simulink model "lab_7_task_3_simulink"  (R2025b)
settings: Solver=ode4  StartTime=0.0  StopTime=10.0  FixedStep=0.0001  RelTol=1e-3
values from neighbouring files (symbols this model uses):
  a = 7093    [lab_7_task_1.m]    (also in lab_7_task_2.m; lab_7_task_3.m; lab_7_task_4.m; project_review.m)
  A_BN0 = eye(3)    [lab_7_task_1.m]    (also in lab_7_task_3.m; lab_7_task_4.m; project_review.m)
  area = [ ... (first row only)    [lab_7_task_3.m]    (also in lab_7_task_4.m; project_review.m)
  e = 0.5    [lab_7_task_1.m]    (also in lab_7_task_2.m; lab_7_task_3.m = 0.00277; lab_7_task_4.m = 0.00277; project_review.m = 0.00277)
  e_sun = deg2rad(23.45)    [lab_7_task_1.m]    (also in lab_7_task_2.m; lab_7_task_3.m; lab_7_task_4.m; project_review.m)
  I = diag([ix iy iz])    [lab_4_task_1.m]    (also in lab_5_task_1.m; lab_5_task_2.m; lab_6_task_1.m = diag([ ix iy iz ]); lab_6_task_2.m = diag([ ix iy iz ]))
  inc = deg2rad(98.27)    [lab_7_task_1.m]    (also in lab_7_task_2.m; lab_7_task_3.m; lab_7_task_4.m; project_review.m = deg2rad(20))
  mu = astroConstants(13)    [lab_7_task_3.m]    (also in lab_7_task_4.m; project_review.m = 398345.74)
  n = sqrt(G*M_e/R^3)    [lab_6_task_1.m]    (also in lab_6_task_2.m; lab_7_task_1.m = sqrt(mu_E/(a^3)); lab_7_task_2.m = sqrt(mu_E/(a^3)); lab_7_task_3.m = sqrt(mu/(a^3)))
  N_B = [ ... (first row only)    [lab_7_task_3.m]    (also in lab_7_task_4.m; project_review.m)
  n_sun = 2*pi / (60*60*24*365)    (= 1.99238499086e-07)    [lab_7_task_1.m]    (also in lab_7_task_2.m; lab_7_task_3.m; lab_7_task_4.m = 1.99102127766e-07; project_review.m = 1.99102127766e-07)
  P = F_e / c    (= 4.52968645764e-06)    [lab_7_task_3.m]    (also in lab_7_task_4.m; project_review.m)
  r_Fi = [ ... (first row only)    [lab_7_task_3.m]    (also in lab_7_task_4.m; project_review.m)
  r_sun = 1.496e8    (= 149600000)    [lab_7_task_1.m]    (also in lab_7_task_2.m; lab_7_task_3.m; lab_7_task_4.m; project_review.m)
  rho_d = [0.1 0.1 0.1 0.1 0.1 0.1      0.1 0.1 0.1 0.1]    [lab_7_task_3.m]    (also in lab_7_task_4.m; project_review.m)
  rho_s = [0.5 0.5 0.5 0.5 0.5 0.5      0.1 0.1 0.1 0.1]    [lab_7_task_3.m]    (also in lab_7_task_4.m; project_review.m)
  TA0 = deg2rad(0)    [lab_7_task_1.m]    (also in lab_7_task_2.m; lab_7_task_3.m; lab_7_task_4.m; project_review.m)
undefined symbols (not defined in the file or in its folder): i
libraries: vec_norm x2, dynamics x1, matrix_library x1
settings Model: VariantFading=off  Creator=nicol  LastModifiedBy=nicol

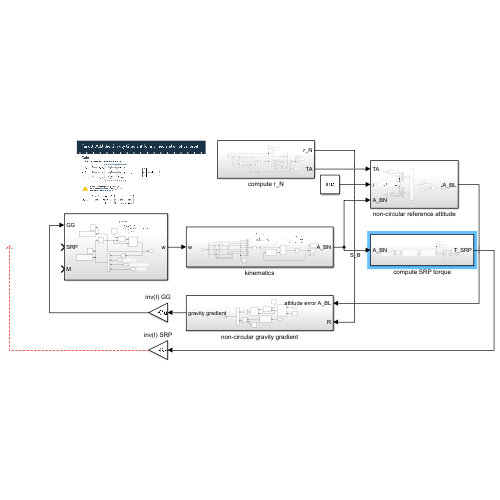
[thumbnail: Simulink's stored preview of the top-level diagram]
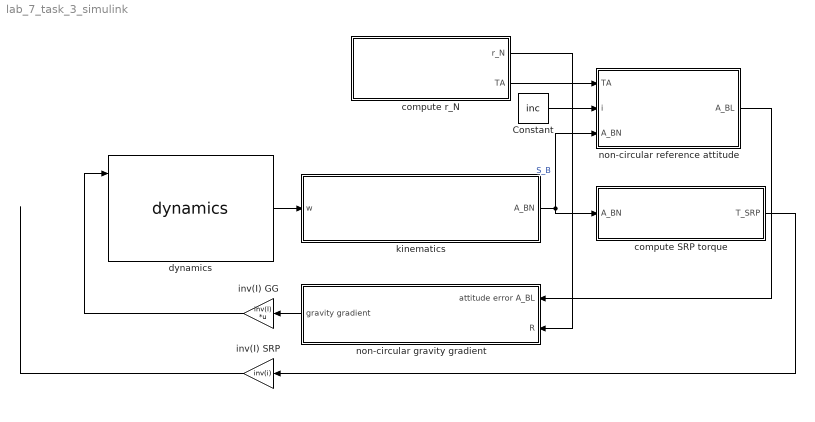
== system lab_7_task_3_simulink ==
  Constant : Constant  Value=inc
  compute SRP torque : Subsystem
  compute r_N : Subsystem
  dynamics : dynamics/dynamics  SystemSampleTime=-1  VariantActivationTime=update diagram  EmptyChoice=off  PassThrough=off  PassThroughVariantControl=(default)  EmptyChoiceVariantControl=(default)  AllowFlexibleInterface=on  Latency=0  AutoFrameSizeCalculation=off
  inv(I) GG : Gain  Gain=inv(I)  Multiplication=Matrix(K*u)
  inv(I) SRP : Gain  Gain=inv(i)
  kinematics : Subsystem
  non-circular gravity gradient : Subsystem
      settings: PortSchema="{\"entries\":[{\"content\":{\"sides\":[{\"content\":{\"connectorIds\":[\"Out1\"]},\"type\":\"ConnectorPlacement.EquallySpacedRectSide\",\"uuid\":\"2a67419a-68c9-4369-a698-e6ac26417455\"},{\"content\":{\"connectorIds\":[\"In1\",\"In2\"],\"side\":\"RIGHT\"},\"type\":\"ConnectorPlacement.EquallySpacedRectSide\",\"uuid\":\"5f3f4c4a-6b79-4b92-8f4c-19ffa36753b2\"},{\"content\":{\"side\":\"TOP\"},\"type\":\"ConnectorPlacement.EquallySpacedRectSide\",\"uuid\":\"22c946b7-ea77-4444-a63c-d5b3d585f671\"}]},\"type\":\"ConnectorPlacement.EquallySpacedConnector\",\"uuid\":\"037c4a72-b28b-418e-a921-9da68dc0cd93\"}],\"packageUris\":[\"http://schema.mathworks.com/mf0/Connector/R2020b\"],\"version\":\"1.0\"}"
  non-circular reference attitude : Subsystem
  wires:
  compute r_N/1(r_N) -> non-circular gravity gradient/2(R)
  Constant/1 -> non-circular reference attitude/2(i)
  inv(I) GG/1 -> dynamics/1
  compute r_N/2(TA) -> non-circular reference attitude/1(TA)
  dynamics/1 -> kinematics/1(w)
  kinematics/1(A_BN) -> compute SRP torque/1(A_BN), non-circular reference attitude/3(A_BN)  "S_B"
  non-circular reference attitude/1(A_BL) -> non-circular gravity gradient/1(attitude error A_BL)
  compute SRP torque/1(T_SRP) -> inv(I) SRP/1
  inv(I) SRP/1 -> ?
  non-circular gravity gradient/1(gravity gradient) -> inv(I) GG/1

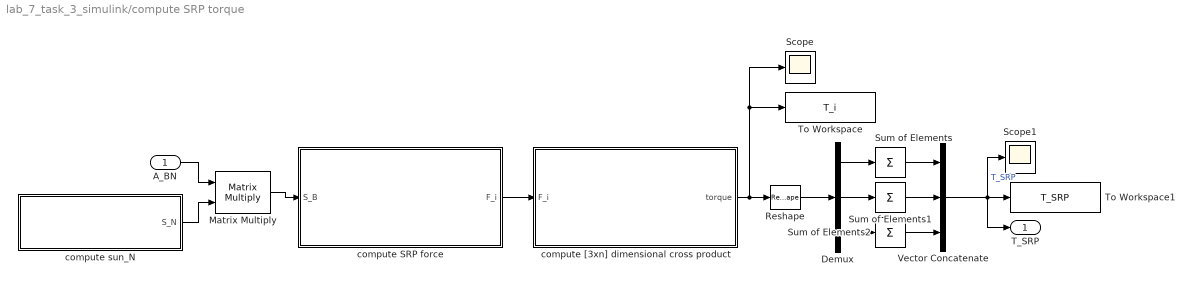
== system lab_7_task_3_simulink/compute SRP torque ==
  A_BN : Inport
  Demux : Demux  Outputs=3
  Matrix Multiply : Product  Multiplication=Matrix(*)
  Reshape : Reshape
  Scope : Scope
      settings: ActiveDisplayYMinimum=-1  ActiveDisplayYMaximum=1  DataLoggingVariableName=ScopeData6
  Scope1 : Scope
      settings: ActiveDisplayYMinimum=-2.7188018298935311E-7  ActiveDisplayYMaximum=4.8585990784799191E-7  DataLoggingVariableName=ScopeData7
  Sum of Elements : Sum  Inputs=+
  Sum of Elements1 : Sum  Inputs=+
  Sum of Elements2 : Sum  Inputs=+
  To Workspace : ToWorkspace  VariableName=T_i  SaveFormat=Timeseries  SampleTime=-1
  To Workspace1 : ToWorkspace  VariableName=T_SRP  SaveFormat=Timeseries  SampleTime=-1
  Vector Concatenate : Concatenate  NumInputs=3
  compute SRP force : Subsystem
  compute [3xn] dimensional cross product : Subsystem
  compute sun_N : Subsystem
  T_SRP : Outport
  wires:
  Matrix Multiply/1 -> compute SRP force/1(S_B)
  compute [3xn] dimensional cross product/1(torque) -> Scope/1, To Workspace/1, Reshape/1
  compute SRP force/1(F_i) -> compute [3xn] dimensional cross product/1(F_i)
  compute sun_N/1(S_N) -> Matrix Multiply/2
  A_BN/1 -> Matrix Multiply/1
  Reshape/1 -> Demux/1
  Demux/3 -> Sum of Elements2/1
  Demux/2 -> Sum of Elements1/1
  Demux/1 -> Sum of Elements/1
  Sum of Elements1/1 -> Vector Concatenate/2
  Sum of Elements/1 -> Vector Concatenate/1
  Sum of Elements2/1 -> Vector Concatenate/3
  Vector Concatenate/1 -> T_SRP/1, Scope1/1, To Workspace1/1  "T_SRP"

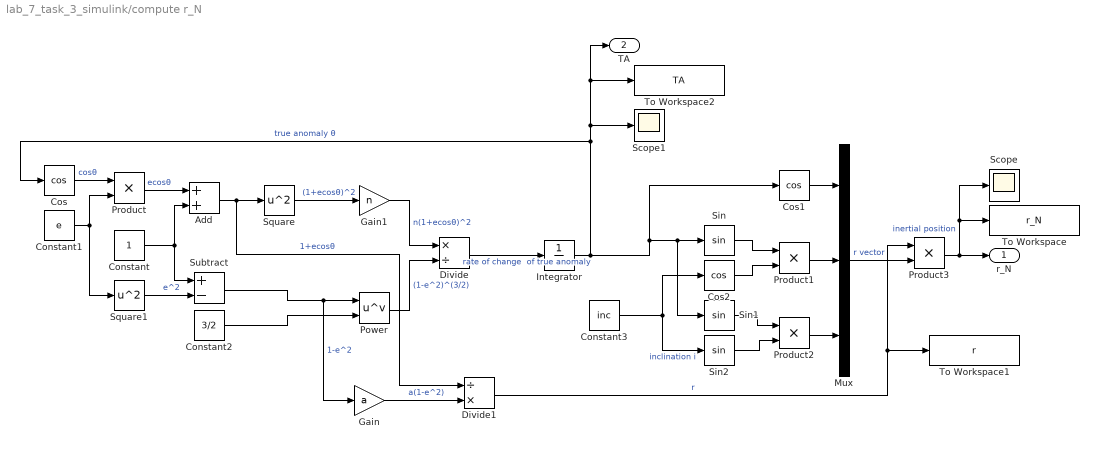
== system lab_7_task_3_simulink/compute r_N ==
  Add : Sum
  Constant : Constant
  Constant1 : Constant  Value=e
  Constant2 : Constant  Value=3/2
  Constant3 : Constant  Value=inc
  Cos : Trigonometry  Operator=cos
  Cos1 : Trigonometry  Operator=cos
  Cos2 : Trigonometry  Operator=cos
  Divide : Product  Inputs=*/
  Divide1 : Product  Inputs=/*
  Gain : Gain  Gain=a
  Gain1 : Gain  Gain=n
  Integrator : Integrator  InitialCondition=TA0
  Mux : Mux  Inputs=3
  Power : Math  Operator=pow
  Product{,1..3} (4 alike) : Product
  Scope : Scope
      settings: ActiveDisplayYMinimum=-1  ActiveDisplayYMaximum=1  DataLoggingVariableName=ScopeData3
  Scope1 : Scope
      settings: ActiveDisplayYMinimum=-1  ActiveDisplayYMaximum=1  DataLoggingVariableName=ScopeData5
  Sin : Trigonometry
  Sin1 : Trigonometry
  Sin2 : Trigonometry
  Square : Math  Operator=square
  Square1 : Math  Operator=square
  Subtract : Sum  Inputs=+-
  To Workspace : ToWorkspace  VariableName=r_N  SaveFormat=Timeseries  SampleTime=-1
  To Workspace1 : ToWorkspace  VariableName=r  SaveFormat=Timeseries  SampleTime=-1
  To Workspace2 : ToWorkspace  VariableName=TA  SaveFormat=Timeseries  SampleTime=-1
  r_N : Outport
  TA : Outport  Port=2
  wires:
  Integrator/1 -> Sin1/1, Sin/1, Cos1/1, To Workspace2/1, TA/1, Scope1/1, Cos/1  "true anomaly θ"
  Add/1 -> Divide1/1, Square/1  "1+ecosθ"
  Square/1 -> Gain1/1  "(1+ecosθ)^2"
  Gain1/1 -> Divide/1  "n(1+ecosθ)^2"
  Sin1/1 -> Product2/1
  Constant/1 -> Subtract/1, Add/2
  Subtract/1 -> Gain/1, Power/1  "1-e^2"
  Product3/1 -> r_N/1, To Workspace/1, Scope/1  "inertial position"
  Constant3/1 -> Cos2/1, Sin2/1  "inclination i"
  Gain/1 -> Divide1/2  "a(1-e^2)"
  Constant2/1 -> Power/2
  Sin2/1 -> Product2/2
  Cos/1 -> Product/1  "cosθ"
  Constant1/1 -> Square1/1, Product/2
  Product/1 -> Add/1  "ecosθ"
  Product2/1 -> Mux/3
  Square1/1 -> Subtract/2  "e^2"
  Divide1/1 -> Product3/1, To Workspace1/1  "r"
  Cos1/1 -> Mux/1
  Mux/1 -> Product3/2  "r vector"
  Power/1 -> Divide/2  "(1-e^2)^(3/2)"
  Product1/1 -> Mux/2
  Divide/1 -> Integrator/1  "rate of change  of true anomaly"
  Sin/1 -> Product1/1
  Cos2/1 -> Product1/2

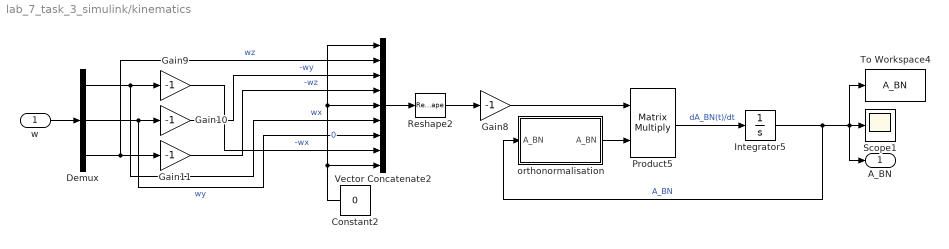
== system lab_7_task_3_simulink/kinematics ==
  w : Inport
  Constant2 : Constant  Value=0
  Demux : Demux  Outputs=3
  Gain{8..11} (4 alike) : Gain  Gain=-1
  Integrator5 : Integrator  InitialCondition=A_BN0
  Product5 : Product  Multiplication=Matrix(*)
  Reshape2 : Reshape  OutputDimensionality=Customize  OutputDimensions=[3,3]
  Scope1 : Scope
      settings: ActiveDisplayYMinimum=-1.2499999998899596  ActiveDisplayYMaximum=1.2499999999877733
  To Workspace4 : ToWorkspace  VariableName=A_BN  SaveFormat=Timeseries  SampleTime=-1
  Vector Concatenate2 : Concatenate  NumInputs=9
  orthonormalisation : Subsystem
  A_BN : Outport
  wires:
  Product5/1 -> Integrator5/1  "dA_BN(t)/dt"
  Gain11/1 -> Vector Concatenate2/4  "-wz"
  Integrator5/1 -> A_BN/1, To Workspace4/1, Scope1/1, orthonormalisation/1(A_BN)  "A_BN"
  Gain8/1 -> Product5/1
  Demux/1 -> Vector Concatenate2/6, Gain9/1  "wx"
  Reshape2/1 -> Gain8/1
  Gain10/1 -> Vector Concatenate2/3  "-wy"
  Demux/2 -> Vector Concatenate2/7, Gain10/1  "wy"
  Vector Concatenate2/1 -> Reshape2/1
  Demux/3 -> Vector Concatenate2/2, Gain11/1  "wz"
  Constant2/1 -> Vector Concatenate2/1, Vector Concatenate2/5, Vector Concatenate2/9  "0"
  Gain9/1 -> Vector Concatenate2/8  "-wx"
  w/1 -> Demux/1
  orthonormalisation/1(" A_BN") -> Product5/2

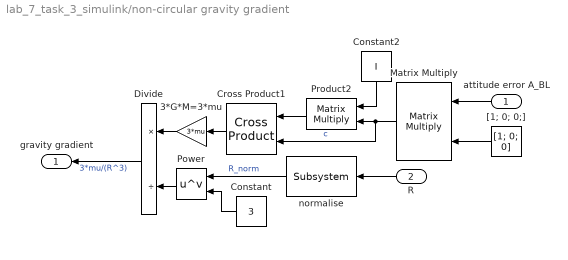
== system lab_7_task_3_simulink/non-circular gravity gradient ==
  attitude error A_BL : Inport
  R : Inport  Port=2
  3*G*M=3*mu : Gain  Gain=3*mu
  Constant : Constant  Value=3
  Constant2 : Constant  Value=I
  Cross Product1 : matrix_library/Cross Product
  Divide : Product  Inputs=*/
  Matrix Multiply : Product  Multiplication=Matrix(*)
  Power : Math  Operator=pow
  Product2 : Product  Multiplication=Matrix(*)
  "[1; 0; 0;]" : Constant  Value=[1; 0; 0]
  normalise : vec_norm/Subsystem  SystemSampleTime=-1  VariantActivationTime=update diagram  EmptyChoice=off  PassThrough=off  PassThroughVariantControl=(default)  EmptyChoiceVariantControl=(default)  AllowFlexibleInterface=on  Latency=0  AutoFrameSizeCalculation=off
  gravity gradient : Outport
  wires:
  Matrix Multiply/1 -> Cross Product1/2, Product2/2  "c"
  attitude error A_BL/1 -> Matrix Multiply/1
  Constant2/1 -> Product2/1
  Cross Product1/1 -> 3*G*M=3*mu/1
  Product2/1 -> Cross Product1/1
  "[1; 0; 0;]"/1 -> Matrix Multiply/2
  3*G*M=3*mu/1 -> Divide/1
  Divide/1 -> gravity gradient/1  "3*mu/(R^3)"
  R/1 -> normalise/1
  Constant/1 -> Power/2
  Power/1 -> Divide/2
  normalise/1 -> Power/1  "R_norm"

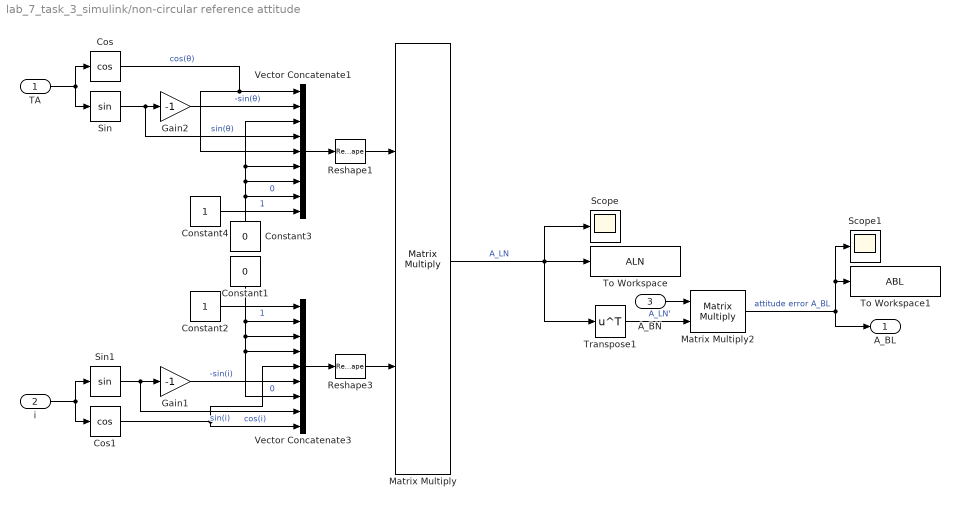
== system lab_7_task_3_simulink/non-circular reference attitude ==
  TA : Inport
  i : Inport  Port=2
  A_BN : Inport  Port=3
  Constant1 : Constant  Value=0
  Constant2 : Constant
  Constant3 : Constant  Value=0
  Constant4 : Constant
  Cos : Trigonometry  Operator=cos
  Cos1 : Trigonometry  Operator=cos
  Gain1 : Gain  Gain=-1
  Gain2 : Gain  Gain=-1
  Matrix Multiply : Product  Multiplication=Matrix(*)
  Matrix Multiply2 : Product  Multiplication=Matrix(*)
  Reshape1 : Reshape  OutputDimensionality=Customize  OutputDimensions=[3,3]
  Reshape3 : Reshape  OutputDimensionality=Customize  OutputDimensions=[3,3]
  Scope : Scope
      settings: ActiveDisplayYMinimum=-1.2499999999912785  ActiveDisplayYMaximum=1.249999999999031  DataLoggingVariableName=ScopeData2
  Scope1 : Scope
      settings: ActiveDisplayYMinimum=-1  ActiveDisplayYMaximum=1  DataLoggingVariableName=ScopeData4
  Sin : Trigonometry
  Sin1 : Trigonometry
  To Workspace : ToWorkspace  VariableName=ALN  SaveFormat=Timeseries  SampleTime=-1
  To Workspace1 : ToWorkspace  VariableName=ABL  SaveFormat=Timeseries  SampleTime=-1
  Transpose1 : Math  Operator=transpose
  Vector Concatenate1 : Concatenate  NumInputs=9
  Vector Concatenate3 : Concatenate  NumInputs=9
  A_BL : Outport
  wires:
  Constant3/1 -> Vector Concatenate1/8, Vector Concatenate1/7, Vector Concatenate1/6, Vector Concatenate1/3  "0"
  TA/1 -> Sin/1, Cos/1
  Gain2/1 -> Vector Concatenate1/2  "-sin(θ)"
  Sin/1 -> Vector Concatenate1/4, Gain2/1  "sin(θ)"
  Matrix Multiply/1 -> Scope/1, Transpose1/1, To Workspace/1  "A_LN"
  Cos/1 -> Vector Concatenate1/5, Vector Concatenate1/1  "cos(θ)"
  Vector Concatenate1/1 -> Reshape1/1
  Constant4/1 -> Vector Concatenate1/9  "1"
  Transpose1/1 -> Matrix Multiply2/2  "A_LN'"
  Reshape1/1 -> Matrix Multiply/1
  Reshape3/1 -> Matrix Multiply/2
  Vector Concatenate3/1 -> Reshape3/1
  Cos1/1 -> Vector Concatenate3/5, Vector Concatenate3/9  "cos(i)"
  Sin1/1 -> Vector Concatenate3/8, Gain1/1  "sin(i)"
  i/1 -> Sin1/1, Cos1/1
  Constant1/1 -> Vector Concatenate3/7, Vector Concatenate3/4, Vector Concatenate3/3, Vector Concatenate3/2  "0"
  Constant2/1 -> Vector Concatenate3/1  "1"
  Gain1/1 -> Vector Concatenate3/6  "-sin(i)"
  A_BN/1 -> Matrix Multiply2/1
  Matrix Multiply2/1 -> Scope1/1, To Workspace1/1, A_BL/1  "attitude error A_BL"

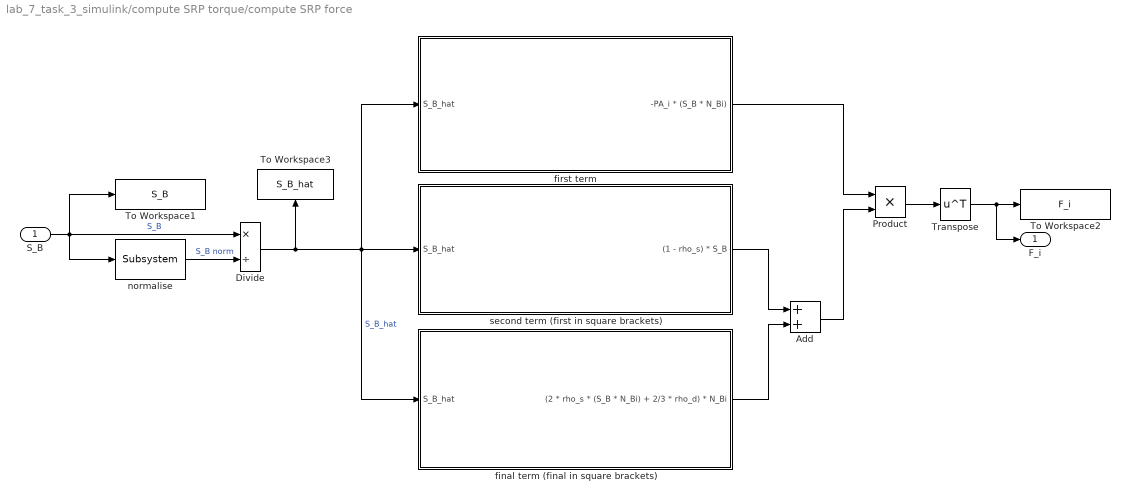
== system lab_7_task_3_simulink/compute SRP torque/compute SRP force ==
  S_B : Inport
  Add : Sum
  Divide : Product  Inputs=*/
  Product : Product
  To Workspace1 : ToWorkspace  VariableName=S_B  SaveFormat=Timeseries  SampleTime=-1
  To Workspace2 : ToWorkspace  VariableName=F_i  SaveFormat=Timeseries  SampleTime=-1
  To Workspace3 : ToWorkspace  VariableName=S_B_hat  SaveFormat=Timeseries  SampleTime=-1
  Transpose : Math  Operator=transpose
  final term (final in square brackets) : Subsystem
  first term : Subsystem
  normalise : vec_norm/Subsystem  SystemSampleTime=-1  VariantActivationTime=update diagram  EmptyChoice=off  PassThrough=off  PassThroughVariantControl=(default)  EmptyChoiceVariantControl=(default)  AllowFlexibleInterface=on  Latency=0  AutoFrameSizeCalculation=off
  second term (first in square brackets) : Subsystem
  F_i : Outport
  wires:
  final term (final in square brackets)/1((2 * rho_s * (S_B * N_Bi) + 2/3 * rho_d) * N_Bi) -> Add/2
  Transpose/1 -> F_i/1, To Workspace2/1
  first term/1(-PA_i * (S_B * N_Bi)) -> Product/1
  Add/1 -> Product/2
  second term (first in square brackets)/1((1 - rho_s) * S_B) -> Add/1
  Product/1 -> Transpose/1
  normalise/1 -> Divide/2  "S_B norm"
  Divide/1 -> second term (first in square brackets)/1(S_B_hat), first term/1(S_B_hat), final term (final in square brackets)/1(S_B_hat), To Workspace3/1  "S_B_hat"
  S_B/1 -> normalise/1, Divide/1, To Workspace1/1  "S_B"

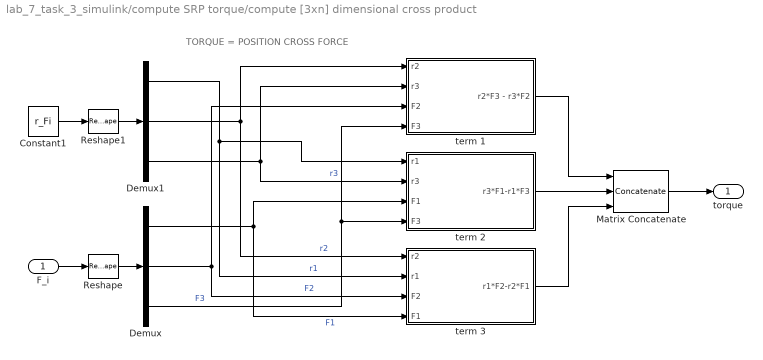
== system lab_7_task_3_simulink/compute SRP torque/compute [3xn] dimensional cross product ==
  note: TORQUE = POSITION CROSS FORCE
  F_i : Inport
  Constant1 : Constant  Value=r_Fi
  Demux : Demux  Outputs=3
  Demux1 : Demux  Outputs=3
  Matrix Concatenate : Concatenate  NumInputs=3  Mode=Multidimensional array  ConcatenateDimension=2
  Reshape : Reshape
  Reshape1 : Reshape
  term 1 : Subsystem
  term 2 : Subsystem
  term 3 : Subsystem
  torque : Outport
  wires:
  term 2/1(r3*F1-r1*F3) -> Matrix Concatenate/2
  Demux1/2 -> term 1/1(r2), term 3/1(r2)  "r2"
  term 3/1(r1*F2-r2*F1) -> Matrix Concatenate/3
  term 1/1(r2*F3 - r3*F2) -> Matrix Concatenate/1
  Demux/2 -> term 1/3(F2), term 3/3(F2)  "F2"
  Demux/3 -> term 1/4(F3), term 2/4(F3)  "F3"
  F_i/1 -> Reshape/1
  Demux1/3 -> term 1/2(r3), term 2/2(r3)  "r3"
  Reshape1/1 -> Demux1/1
  Constant1/1 -> Reshape1/1
  Demux/1 -> term 2/3(F1), term 3/4(F1)  "F1"
  Demux1/1 -> term 3/2(r1), term 2/1(r1)  "r1"
  Reshape/1 -> Demux/1
  Matrix Concatenate/1 -> torque/1

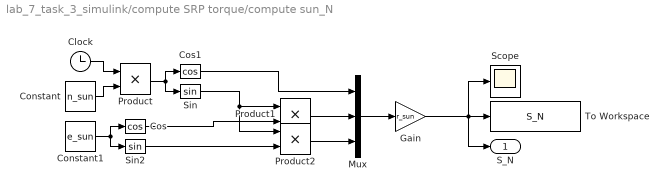
== system lab_7_task_3_simulink/compute SRP torque/compute sun_N ==
  Clock : Clock
  Constant : Constant  Value=n_sun
  Constant1 : Constant  Value=e_sun
  Cos : Trigonometry  Operator=cos
  Cos1 : Trigonometry  Operator=cos
  Gain : Gain  Gain=r_sun
  Mux : Mux  Inputs=3
  Product : Product
  Product1 : Product
  Product2 : Product
  Scope : Scope
      settings: ActiveDisplayYMinimum=-1.8699999999999996E+7  ActiveDisplayYMaximum=1.683E+8
  Sin : Trigonometry
  Sin2 : Trigonometry
  To Workspace : ToWorkspace  VariableName=S_N  SaveFormat=Timeseries  SampleTime=-1
  S_N : Outport
  wires:
  Constant/1 -> Product/2
  Clock/1 -> Product/1
  Product/1 -> Sin/1, Cos1/1
  Constant1/1 -> Sin2/1, Cos/1
  Cos1/1 -> Mux/1
  Product1/1 -> Mux/2
  Product2/1 -> Mux/3
  Sin/1 -> Product2/1, Product1/1
  Cos/1 -> Product1/2
  Sin2/1 -> Product2/2
  Gain/1 -> S_N/1, Scope/1, To Workspace/1
  Mux/1 -> Gain/1

== system lab_7_task_3_simulink/kinematics/orthonormalisation ==
  A_BN : Inport
  Gain : Gain  Gain=3/2
  Gain1 : Gain  Gain=1/2
  Matrix Multiply1 : Product  Inputs=3  Multiplication=Matrix(*)
  Subtract : Sum  Inputs=+-
  Transpose1 : Math  Operator=transpose
  " A_BN" : Outport
  wires:
  Gain/1 -> Subtract/1
  Transpose1/1 -> Matrix Multiply1/2
  Matrix Multiply1/1 -> Gain1/1
  Gain1/1 -> Subtract/2
  Subtract/1 -> " A_BN"/1
  A_BN/1 -> Matrix Multiply1/1, Gain/1, Transpose1/1, Matrix Multiply1/3

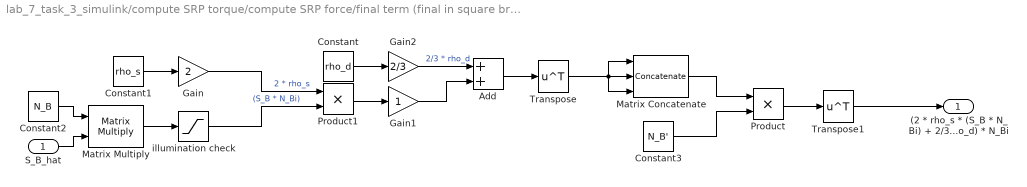
== system lab_7_task_3_simulink/compute SRP torque/compute SRP force/final term (final in square brackets) ==
  S_B_hat : Inport
  Add : Sum
  Constant : Constant  Value=rho_d
  Constant1 : Constant  Value=rho_s
  Constant2 : Constant  Value=N_B
  Constant3 : Constant  Value=N_B'
  Gain : Gain  Gain=2
  Gain1 : Gain
  Gain2 : Gain  Gain=2/3
  Matrix Concatenate : Concatenate  NumInputs=3  Mode=Multidimensional array
  Matrix Multiply : Product  Multiplication=Matrix(*)
  Product : Product
  Product1 : Product
  Transpose : Math  Operator=transpose
  Transpose1 : Math  Operator=transpose
  illumination check : Saturate  UpperLimit=inf  LowerLimit=0
  (2 * rho_s * (S_B * N_Bi) + 2/3 * rho_d) * N_Bi : Outport
  wires:
  Constant1/1 -> Gain/1
  Product1/1 -> Gain1/1
  Gain1/1 -> Add/2
  Transpose1/1 -> (2 * rho_s * (S_B * N_Bi) + 2/3 * rho_d) * N_Bi/1
  Constant3/1 -> Product/2
  Transpose/1 -> Matrix Concatenate/3, Matrix Concatenate/1, Matrix Concatenate/2
  S_B_hat/1 -> Matrix Multiply/2
  Constant2/1 -> Matrix Multiply/1
  Matrix Multiply/1 -> illumination check/1
  Gain/1 -> Product1/1  "2 * rho_s"
  Constant/1 -> Gain2/1
  Gain2/1 -> Add/1  "2/3 * rho_d"
  Add/1 -> Transpose/1
  Matrix Concatenate/1 -> Product/1
  Product/1 -> Transpose1/1
  illumination check/1 -> Product1/2  "(S_B * N_Bi)"

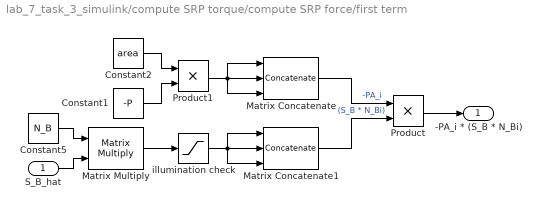
== system lab_7_task_3_simulink/compute SRP torque/compute SRP force/first term ==
  S_B_hat : Inport
  Constant1 : Constant  Value=-P
  Constant2 : Constant  Value=area
  Constant5 : Constant  Value=N_B
  Matrix Concatenate : Concatenate  NumInputs=3  Mode=Multidimensional array  ConcatenateDimension=2
  Matrix Concatenate1 : Concatenate  NumInputs=3  Mode=Multidimensional array  ConcatenateDimension=2
  Matrix Multiply : Product  Multiplication=Matrix(*)
  Product : Product
  Product1 : Product
  illumination check : Saturate  UpperLimit=inf  LowerLimit=0
  -PA_i * (S_B * N_Bi) : Outport
  wires:
  Product/1 -> -PA_i * (S_B * N_Bi)/1
  S_B_hat/1 -> Matrix Multiply/2
  Constant5/1 -> Matrix Multiply/1
  Constant2/1 -> Product1/1
  Constant1/1 -> Product1/2
  Product1/1 -> Matrix Concatenate/1, Matrix Concatenate/3, Matrix Concatenate/2
  Matrix Concatenate/1 -> Product/1  "-PA_i"
  illumination check/1 -> Matrix Concatenate1/3, Matrix Concatenate1/1, Matrix Concatenate1/2
  Matrix Concatenate1/1 -> Product/2  "(S_B * N_Bi)"
  Matrix Multiply/1 -> illumination check/1

== system lab_7_task_3_simulink/compute SRP torque/compute SRP force/second term (first in square brackets) ==
  S_B_hat : Inport
  Constant1 : Constant
  Constant2 : Constant  Value=rho_s
  Matrix Multiply : Product  Multiplication=Matrix(*)
  Subtract : Sum  Inputs=+-
  Transpose : Math  Operator=transpose
  (1 - rho_s) * S_B : Outport
  wires:
  Constant2/1 -> Subtract/2
  Constant1/1 -> Subtract/1
  Matrix Multiply/1 -> (1 - rho_s) * S_B/1
  Subtract/1 -> Matrix Multiply/1
  S_B_hat/1 -> Transpose/1
  Transpose/1 -> Matrix Multiply/2

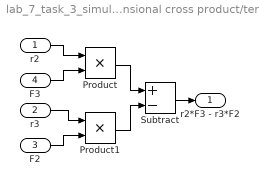
== system lab_7_task_3_simulink/compute SRP torque/compute [3xn] dimensional cross product/term 1 ==
  r2 : Inport
  r3 : Inport  Port=2
  F2 : Inport  Port=3
  F3 : Inport  Port=4
  Product : Product
  Product1 : Product
  Subtract : Sum  Inputs=+-
  r2*F3 - r3*F2 : Outport
  wires:
  F3/1 -> Product/2
  Product/1 -> Subtract/1
  F2/1 -> Product1/2
  r2/1 -> Product/1
  Product1/1 -> Subtract/2
  Subtract/1 -> r2*F3 - r3*F2/1
  r3/1 -> Product1/1

== system lab_7_task_3_simulink/compute SRP torque/compute [3xn] dimensional cross product/term 2 ==
  r1 : Inport
  r3 : Inport  Port=2
  F1 : Inport  Port=3
  F3 : Inport  Port=4
  Product : Product
  Product1 : Product
  Subtract : Sum  Inputs=+-
  r3*F1-r1*F3 : Outport
  wires:
  F3/1 -> Product1/2
  Product1/1 -> Subtract/2
  Product/1 -> Subtract/1
  F1/1 -> Product/2
  r3/1 -> Product/1
  Subtract/1 -> r3*F1-r1*F3/1
  r1/1 -> Product1/1

== system lab_7_task_3_simulink/compute SRP torque/compute [3xn] dimensional cross product/term 3 ==
  r2 : Inport
  r1 : Inport  Port=2
  F2 : Inport  Port=3
  F1 : Inport  Port=4
  Product : Product
  Product1 : Product
  Subtract : Sum  Inputs=+-
  r1*F2-r2*F1 : Outport
  wires:
  F1/1 -> Product1/2
  r1/1 -> Product/1
  Product1/1 -> Subtract/2
  F2/1 -> Product/2
  Product/1 -> Subtract/1
  r2/1 -> Product1/1
  Subtract/1 -> r1*F2-r2*F1/1
